simulink model "serialecho"  (R2022b)
settings: Solver=FixedStepDiscrete  StartTime=0.0  StopTime=inf  FixedStep=0.001  RelTol=1e-3
libraries: teensy_lib x3
settings Model: Creator=LabUser  LastModifiedBy=LabUser
settings OptimizationCC: EnhancedBackFolding=on  PassReuseOutputArgsAs=Individual arguments  ZeroExternalMemoryAtStartup=off  ZeroInternalMemoryAtStartup=off  OptimizeBlockOrder=speed  DifferentSizesBufferReuse=on  OptimizationCustomize=off  EfficientTunableParamExpr=on
settings DebuggingCC: ParameterTunabilityLossMsg=error
settings HardwareCC: ProdBitPerPointer=32  ProdBitPerSizeT=32  ProdBitPerPtrDiffT=32  ProdLargestAtomicInteger=Long  ProdLargestAtomicFloat=Double  ProdWordSize=32  ProdHWDeviceType=ARM Compatible->ARM Cortex-M
settings SFSimCC: MATLABDynamicMemAlloc=off
settings RTWCC: Description=Teensy ERT Target  SystemTargetFile=teensy_ert.tlc  TemplateMakefile=teensy_ert.tmf  TargetLang=C++
settings CodeAppCC: ForceParamTrailComments=on  IgnoreCustomStorageClasses=off  OperatorAnnotations=on  SimulinkDataObjDesc=on  SFDataObjDesc=on  InsertBlockDesc=on
settings STFCustomTargetCC: TargetLibSuffix=.a  TargetLangStandard=C++11 (ISO)  MultiwordLength=256  GenerateSampleERTMain=on  CombineOutputUpdateFcns=on  ERTCustomFileBanners=on  SupportContinuousTime=off  SupportNonInlinedSFcns=off  RemoveResetFunc=on  MATLABClassNameForMDSCustomization=Simulink.SoftwareTarget.ERTCustomization  CPPClassGenCompliant=on  SystemTargetFile=teensy_ert.tlc
settings ERTTargetCC: TargetLangStandard=C++11 (ISO)  GenerateSampleERTMain=on  ParMdlRefBuildCompliant=off  CompOptLevelCompliant=off  ConcurrentExecutionCompliant=off  ModelStepFunctionPrototypeControlCompliant=off  UseToolchainInfoCompliant=off  ExtModeTransport=1  ExtModeMexFile=ext_serial_win32_comm  ExtModeMexArgs=0 5 4000000  ERTCustomFileTemplate=teensy_ert_file_process.tlc

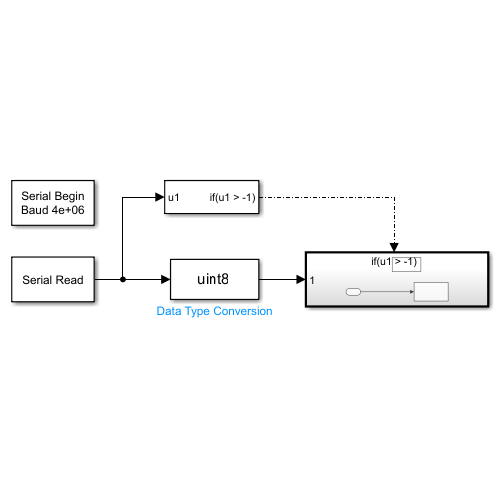
[thumbnail: Simulink's stored preview of the top-level diagram]
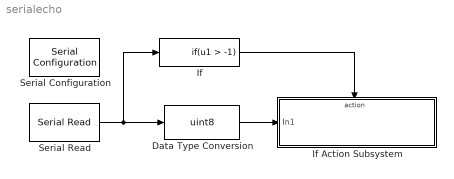
== system serialecho ==
  Data Type Conversion : DataTypeConversion  OutDataTypeStr=uint8  SaturateOnIntegerOverflow=off  RndMeth=Floor
  If : If  IfExpression=u1 > -1  ShowElse=off
  If Action Subsystem : Subsystem  TreatAsAtomicUnit=on
  Serial Configuration : teensy_lib/Serial Configuration  SParameter1=Serial  SParameter2=4000000
  Serial Read : teensy_lib/Serial Read  SParameter1=Serial  SampleTime=-1
  wires:
  Serial Read/1 -> If/1, Data Type Conversion/1
  If/1 -> If Action Subsystem/Action
  Data Type Conversion/1 -> If Action Subsystem/1(In1)

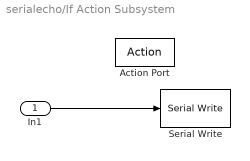
== system serialecho/If Action Subsystem ==
  In1 : Inport
  Action Port : ActionPort  ActionPortLabel=if(u1 > -1)
  Serial Write : teensy_lib/Serial Write  SParameter1=Serial  SampleTime=-1
  wires:
  In1/1 -> Serial Write/1
